simulink model "Events1"  (Simulink 10.0)
settings: Solver=ode45  StartTime=0.0  StopTime=10.0  RelTol=1e-3  EnableMultiTasking=on
settings Model: Creator=scaife  LastModifiedBy=hbourbou  ExtModeAutoUpdateStatusClock=off
settings DataIOCC: LimitDataPoints=on  SignalLoggingSaveFormat=ModelDataLogs  SignalLoggingName=sigsOut
settings DebuggingCC: SaveWithParameterizedLinksMsg=none  SignalResolutionControl=TryResolveAllWithWarning  MultiTaskDSMMsg=warning  MultiTaskCondExecSysMsg=none
settings HardwareCC: TargetUnknown=on
settings SFSimCC: SimParseCustomCode=off
settings ConfigComp: CovExternalEMLEnable=off

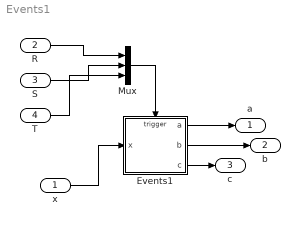
== system Events1 ==
  x : Inport
  R : Inport  Port=2
  S : Inport  Port=3
  T : Inport  Port=4
  Events1 : Stateflow chart  TreatAsAtomicUnit=on
  Mux : Mux  Inputs=3
  a : Outport
  b : Outport  Port=2
  c : Outport  Port=3
  wires:
  x/1 -> Events1/1(x)
  Mux/1 -> Events1/Trigger
  R/1 -> Mux/1
  S/1 -> Mux/2
  T/1 -> Mux/3
  Events1/1(a) -> a/1
  Events1/2(b) -> b/1
  Events1/3(c) -> c/1

== stateflow chart Events1 ==
  state A [parallel]
    settings: executionOrder=1
    state A2
      state A2a/
        en:a=x+3
      state A2b/
        en:a=x+4
      (default) -> A2a
      A2a -> A2b : S/send(S1,B)
      A2b -> A2a : R/send(R1,B)
    state A1
      state A1a/
        en:a=x+1
      state A1b/
        en:a++;
      (default) -> A1a
      A1a -> A1b : S/send(S1,B)
      A1b -> A1a : R/send(R1,B)
    (default) -> A1
    A1 -> A2 : T/send(T1,B)
    A2 -> A1 : T/send(T1,B)
  state B [parallel]
    settings: executionOrder=2
    state B2
      state B2a/
        en:b=x+7
      state B2b/
        en:b=x+8
      (default) -> B2a
      B2a -> B2b : S1
      B2b -> B2a : R1
    state B1
      state B1a/
        en:b=x+5
      state B1b/
        en:b=x+6
      (default) -> B1a
      B1a -> B1b : S1
      B1b -> B1a : R1
    (default) -> B1
    B1 -> B2 : T1/c++
    B2 -> B1 : T1/c++
  data: a output int32; x input int32; b output int32; c output int32
  events: R1 local EITHER_EDGE_EVENT; S1 local EITHER_EDGE_EVENT; T1 local EITHER_EDGE_EVENT; R input EITHER_EDGE_EVENT; S input EITHER_EDGE_EVENT; T input EITHER_EDGE_EVENT
